simulink model "ClosedLoopTestMPC"  (R2025b)
settings: Solver=FixedStepAuto  StartTime=0.0  StopTime=60  FixedStep=Ts  MaxStep=0.015  RelTol=1e-3
StopFcn:
  | stopHeli_allTasks
  | daqreset
model workspace: external: MAT-File (data not in the file)
undefined symbols (not defined in the file or in its folder): A_bar, DAC_lim_u, DiscIntNeverNeededParam, Discrete, ElevAxisData, l, N, nu, nx, PitchAxisData, Q, q, QN, R_kalman, Time, Ts, U_e_real, x0, x0_bar
libraries: ctrlSharedLib x1, sldrtlib x1
settings Model: Creator=msciola  LastModifiedBy=leeta
settings SolverCC: AlgebraicLoopSolver=TrustRegion
settings DebuggingCC: UnconnectedInputMsg=warning  UnconnectedOutputMsg=warning  UnconnectedLineMsg=warning
settings ModelReferenceCC: EnableRefExpFcnMdlSchedulingChecks=on
settings SFSimCC: CustomCodeUndefinedFunction=UseInterfaceOnly
settings RTWCC: GPUComputeCapability=3.5

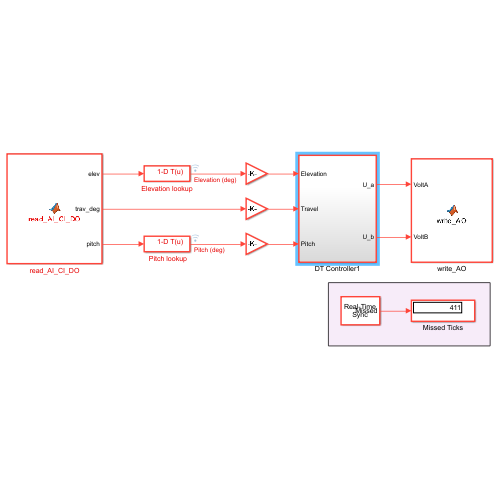
[thumbnail: Simulink's stored preview of the top-level diagram]
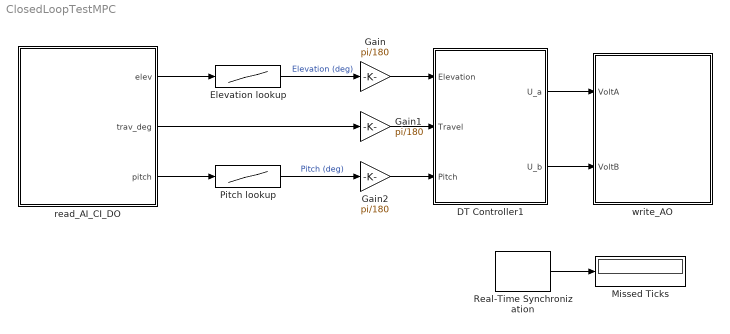
== system ClosedLoopTestMPC ==
  " Pitch lookup" : Lookup_n-D  NumberOfTableDimensions=1  LookupTableObject=PitchAxisData  BreakpointsForDimension1=PitchAxisData.Var2  Table=PitchAxisData.Var1  InternalRulePriority=Speed  RndMeth=Simplest
  DT Controller1 : Subsystem
  Elevation lookup : Lookup_n-D  NumberOfTableDimensions=1  LookupTableObject=PitchAxisData  BreakpointsForDimension1=ElevAxisData.Var2  Table=ElevAxisData.Var1  InternalRulePriority=Speed  RndMeth=Simplest
  Gain : Gain  Gain=pi/180
  Gain1 : Gain  Gain=pi/180
  Gain2 : Gain  Gain=pi/180
  Missed Ticks : Display
  Real-Time Synchronization : sldrtlib/Real-Time Synchronization  SampleTime=Ts  MaxMissedTicks=inf  ShowMissedTicks=on  YieldWhenWaiting=off
  read_AI_CI_DO : MATLAB Function  TreatAsAtomicUnit=on
  write_AO : MATLAB Function  TreatAsAtomicUnit=on
  wires:
  Real-Time Synchronization/1 -> Missed Ticks/1
  DT Controller1/2(U_b) -> write_AO/2(VoltB)
  DT Controller1/1(U_a) -> write_AO/1(VoltA)
  " Pitch lookup"/1 -> Gain2/1  "Pitch (deg)"
  Elevation lookup/1 -> Gain/1  "Elevation (deg)"
  read_AI_CI_DO/2(trav_deg) -> Gain1/1
  read_AI_CI_DO/1(elev) -> Elevation lookup/1
  Gain1/1 -> DT Controller1/2(Travel)
  Gain/1 -> DT Controller1/1(Elevation)
  Gain2/1 -> DT Controller1/3(Pitch)
  read_AI_CI_DO/3(pitch) -> " Pitch lookup"/1

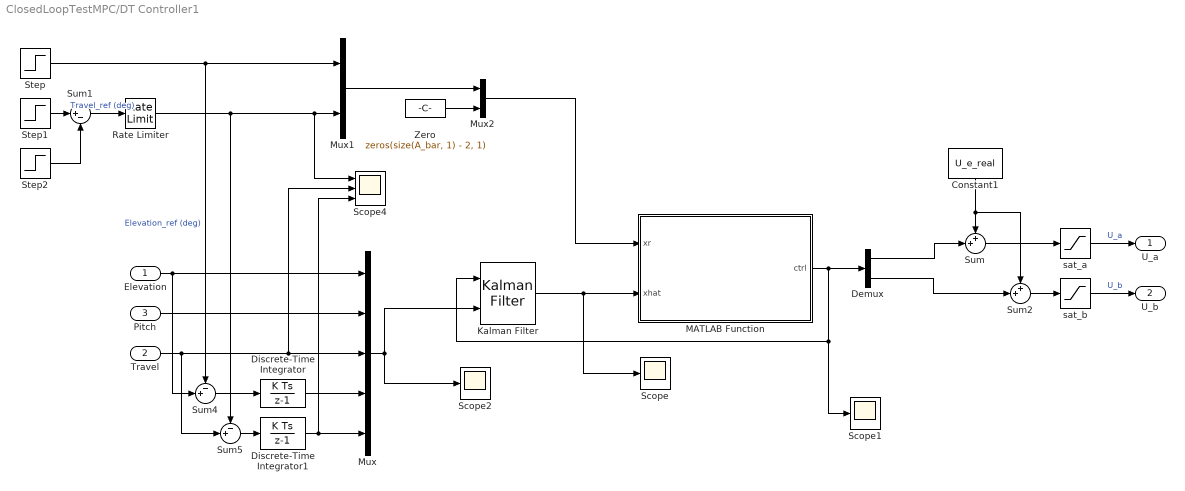
== system ClosedLoopTestMPC/DT Controller1 ==
  Elevation : Inport
  Travel : Inport  Port=2
  Pitch : Inport  Port=3
  Constant1 : Constant  Value=U_e_real
  Demux : Demux  Outputs=2
  Discrete-Time Integrator : DiscreteIntegrator  SampleTime=Ts  ICPrevOutput=DiscIntNeverNeededParam  ICPrevScaledInput=DiscIntNeverNeededParam
  Discrete-Time Integrator1 : DiscreteIntegrator  SampleTime=Ts  ICPrevOutput=DiscIntNeverNeededParam  ICPrevScaledInput=DiscIntNeverNeededParam
  Kalman Filter : ctrlSharedLib/Kalman Filter  TimeDomain=Discrete-Time  UseCurrentEstimator=on  ModelSource=LTI State-Space Variable  ModelSourceVariable=sysdt_bar  A=0.95  B=1  C=1  D=0  NumberOfStates=1  NumberOfInputs=1  NumberOfOutputs=1  InitialEstimateSource=Dialog  X0=x0_bar  P0=10  UseK=off  UseGH=off  NumberOfProcessNoiseInputs=1  G=1  TimeInvariantG=on  H=0  TimeInvariantH=on  Q=1  TimeInvariantQ=on  R=R_kalman  TimeInvariantR=on  N=0  TimeInvariantN=on  AddInputPort=on  AddEnablePort=off  OutputEstimatedY=off  OutputP=off  Ts=-1
  MATLAB Function : MATLAB Function  TreatAsAtomicUnit=on
  Mux : Mux  Inputs=5
  Mux1 : Mux  Inputs=2
  Mux2 : Mux  Inputs=2
  Rate Limiter : RateLimiter  RisingSlewLimit=.5  FallingSlewLimit=-.5  SampleTimeMode=inherited
  Scope : Scope
      settings: ActiveDisplayYMinimum=-62.544393071790253  ActiveDisplayYMaximum=128.86526471159308  DataLoggingVariableName=ScopeData3
  Scope1 : Scope
      settings: ActiveDisplayYMinimum=-1.3821336696475406  ActiveDisplayYMaximum=7.2617510806537968  DataLoggingVariableName=ScopeData4
  Scope2 : Scope
      settings: ActiveDisplayYMinimum=-53.331174165811589  ActiveDisplayYMaximum=47.899230632174024  DataLoggingVariableName=ScopeData3
  Scope4 : Scope  NumInputPorts=3
      settings: ActiveDisplayYMinimum=-183.28076160318139  ActiveDisplayYMaximum=95.493160613464582
  Step : Step  Time=0  Before=x0(1)  After=0  SampleTime=Ts
  Step1 : Step  Time=10  Before=x0(2)  After=deg2rad(180)  SampleTime=Ts
  Step2 : Step  Time=30  Before=x0(3)  After=deg2rad(180)  SampleTime=Ts
  Sum : Sum  Inputs=++|
  Sum1 : Sum  Inputs=|+-
  Sum2 : Sum  Inputs=++|
  Sum4 : Sum  Inputs=-+|
  Sum5 : Sum  Inputs=-+|
  Zero : Constant  Value=zeros(size(A_bar, 1) - 2, 1)
  sat_a : Saturate  UpperLimit=DAC_lim_u  LowerLimit=0
  sat_b : Saturate  UpperLimit=DAC_lim_u  LowerLimit=0
  U_a : Outport
  U_b : Outport  Port=2
  wires:
  sat_b/1 -> U_b/1  "U_b"
  sat_a/1 -> U_a/1  "U_a"
  Kalman Filter/1 -> Scope/1, MATLAB Function/2(xhat)
  MATLAB Function/1(ctrl) -> Scope1/1, Kalman Filter/1, Demux/1
  Demux/1 -> Sum/2
  Demux/2 -> Sum2/2
  Sum/1 -> sat_a/1
  Sum2/1 -> sat_b/1
  Constant1/1 -> Sum2/1, Sum/1
  Zero/1 -> Mux2/2
  Mux2/1 -> MATLAB Function/1(xr)
  Mux/1 -> Kalman Filter/2, Scope2/1
  Elevation/1 -> Sum4/2, Mux/1
  Step2/1 -> Sum1/2
  Step/1 -> Sum4/1, Mux1/1  "Elevation_ref (deg)"
  Rate Limiter/1 -> Sum5/1, Scope4/1, Mux1/2
  Sum5/1 -> Discrete-Time Integrator1/1
  Mux1/1 -> Mux2/1
  Discrete-Time Integrator1/1 -> Scope4/3, Mux/5
  Step1/1 -> Sum1/1
  Discrete-Time Integrator/1 -> Mux/4
  Travel/1 -> Sum5/2, Mux/3, Scope4/2
  Sum4/1 -> Discrete-Time Integrator/1
  Pitch/1 -> Mux/2
  Sum1/1 -> Rate Limiter/1  "Travel_ref (deg)"

== matlab function ClosedLoopTestMPC/DT Controller1/MATLAB Function ==
  data: xr input double size=nx; xhat input double size=nx; ctrl output double size=nu; l parameter; u parameter; q parameter; Q parameter; QN parameter; nx parameter; nu parameter; N parameter
function ctrl = mpc_step(xr, xhat, l, u, q, Q, QN, nx, nu, N)

    coder.extrinsic('emosqp')
    % Update OSQP problem
    % Update initial state

    l(1:nx) = -xhat;
    u(1:nx) = -xhat;

    % Update cost for variable xr
    q = [repmat(-Q*xr, N, 1); -QN*xr; zeros(N*nu, 1)];

    emosqp('update_bounds', l, u);
    emosqp('update_lin_cost', q);

    [x, ~, ~, ~, ~] = emosqp('solve'); 

    ctrl = x((N+1)*nx+1:(N+1)*nx+nu);
    % ctrl(1) = ctrl(1) + U_e;
    % ctrl(2) = ctrl(2) + U_e;
end

== matlab function ClosedLoopTestMPC/write_AO ==
  data: VoltA input; VoltB input
function write_AO(VoltA,VoltB)
% The functions from the NI library to write outpus cannot be compiled 
% and we need to use the coder.extrinsic.
% Functions in common to all  
coder.extrinsic('NI_DAQmxCreateTask','NI_DAQmxStartTask', 'assignin');
% Functions to write AO
coder.extrinsic('NI_DAQmxCreateAOVoltageChan','NI_DAQmxWriteAnalogF64',...
    'daq.ni.NIDAQmx.DAQmx_Val_Volts');
%% Configuration
% Specify channel
channelNameAO = {'myDAQ1/ao0','myDAQ1/ao1'};
% make the taskhandle persistent
persistent  taskHandleAO 
% Create and start tasks for each channel
if isempty(taskHandleAO)
    taskHandleAO = NI_DAQmxCreateTask;
    NI_DAQmxCreateAOVoltageChan(taskHandleAO, channelNameAO{1})
    NI_DAQmxCreateAOVoltageChan(taskHandleAO, channelNameAO{2})
    NI_DAQmxStartTask(taskHandleAO);
    assignin('base','taskHandleAO',taskHandleAO);
end
%% Write Digital output
NI_DAQmxWriteAnalogF64(taskHandleAO,[VoltA,VoltB]);
end

== matlab function ClosedLoopTestMPC/read_AI_CI_DO ==
  data: elev output; trav_deg output; pitch output
function [elev,trav_deg,pitch] = read_AI_CI_DO()
% The functions from the NI library to read and write inputs and outpus 
% cannot be compiled and we need to use the coder.extrinsic.
% Functions in common to all 
coder.extrinsic('NI_DAQmxCreateTask','NI_DAQmxStartTask','assignin');
%Functions to read AI
coder.extrinsic('daq.ni.NIDAQmx.DAQmx_Val_Diff','NI_DAQmxCreateAIVoltageChan',...
    'NI_DAQmxReadAnalogF64');
%Functions to read CI
coder.extrinsic('NI_DAQmxCreateCILinEncoderChan','NI_DAQmxReadCounterScalarF64',... 
    'daq.ni.NIDAQmx.DAQmx_Val_X1','daq.ni.NIDAQmx.DAQmx_Val_Ticks');
%Functions to write DO
coder.extrinsic('NI_DAQmxWriteDigitalLines','NI_DAQmxCreateDOChan');

%% Configuration
% Specify channels
channelNameAI = {'myDAQ1/ai0','myDAQ1/ai1'};
channelNameCI = 'myDAQ1/ctr0';
channelNamesDO = {'myDAQ1/Port0/Line5', 'myDAQ1/Port0/Line6','myDAQ1/Port0/Line7'};

% Initialize variables for MATLAB Function block to work
elev = 0;
pitch = 0;
numChannels = 1;
trav = zeros(1, numChannels);
y = zeros(1, numChannels);
% make the taskhandle for each channel persistent
persistent taskHandleAI taskHandleCI taskHandleDO
% Create and start tasks for each channel
if isempty(taskHandleAI)
    taskHandleAI = NI_DAQmxCreateTask;
    NI_DAQmxCreateAIVoltageChan(taskHandleAI, channelNameAI{1}, daq.ni.NIDAQmx.DAQmx_Val_Diff, -10, 10)
    NI_DAQmxCreateAIVoltageChan(taskHandleAI, channelNameAI{2}, daq.ni.NIDAQmx.DAQmx_Val_Diff, -10, 10)
    NI_DAQmxStartTask(taskHandleAI);
    assignin('base','taskHandleAI',taskHandleAI);
end
if isempty(taskHandleCI)
    taskHandleCI = NI_DAQmxCreateTask;
    NI_DAQmxCreateCILinEncoderChan( taskHandleCI, channelNameCI, daq.ni.NIDAQmx.DAQmx_Val_X1, daq.ni.NIDAQmx.DAQmx_Val_Ticks, 1); % Check X4 (Labview) or X1 with Bryn
    NI_DAQmxStartTask(taskHandleCI)
    assignin('base','taskHandleCI',taskHandleCI);
end
if isempty (taskHandleDO)
    taskHandleDO = NI_DAQmxCreateTask;
    for ii = 1:numel(channelNamesDO)
        NI_DAQmxCreateDOChan(taskHandleDO, channelNamesDO{ii});
    end
    %numChannelsDO = NI_DAQmxGetWriteNumChans(taskHandleDO);
    NI_DAQmxStartTask(taskHandleDO)
    assignin('base','taskHandleDO',taskHandleDO);
end
%% Read and write channels
% Write the digital outputs
outputData = [0 1 0];
NI_DAQmxWriteDigitalLines(taskHandleDO, outputData);
% Read analog inputs (elevation and pitch angles)
data = NI_DAQmxReadAnalogF64(taskHandleAI,1,2);
elev = data(1);
pitch = data(2);

% Read the counter encoder input (tavel angle)
y = NI_DAQmxReadCounterScalarF64(taskHandleCI);
% To avoid insignificant numbers in the reading
if y> 2^31
    y = y- 2^32;
end
% Transform the encoder reading into angle degrees between 0 and 360
 trav_deg = y*360/500;
